simulink model "Lab_6_Hydraulic_Assist_ibrahim"  (R2018b)
settings: Solver=VariableStepAuto  StartTime=0.0  StopTime=5  MaxStep=0.0001  RelTol=1e-3
undefined symbols (not defined in the file): a_neg, A_neg, A_pos, a_pos, ar_neg, Ar_neg, Ar_pos, ar_pos, F_human_max, F_rated_wheel, k, k_dec, kr, kr_dec, Lever_ratio, P_servo_max, R_master, R_servo, R_wheel, s_rated_wheel, V_initial
libraries: nesl_utility x16, sdl_lib x9, fl_lib x8, eeGeneralControl x1, SignalEditorBlockLib x1
settings Model: Creator=AHMED MOHSEN  LastModifiedBy=AHMED MOHSEN
settings DataIOCC: ReturnWorkspaceOutputs=on
settings DebuggingCC: UnconnectedInputMsg=none  UnconnectedOutputMsg=none  UnconnectedLineMsg=none
settings ModelReferenceCC: EnableRefExpFcnMdlSchedulingChecks=off
settings RTWCC: Description=Generic Real-Time Target

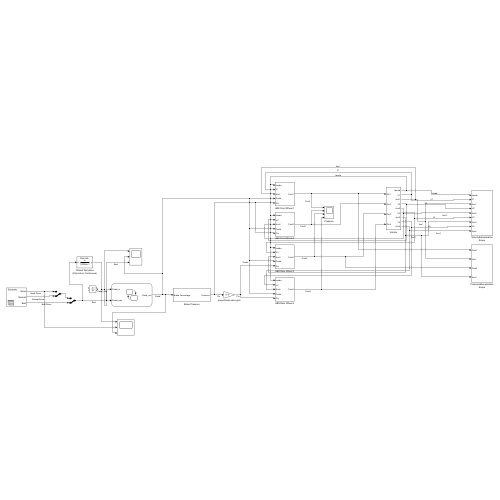
[thumbnail: Simulink's stored preview of the top-level diagram]
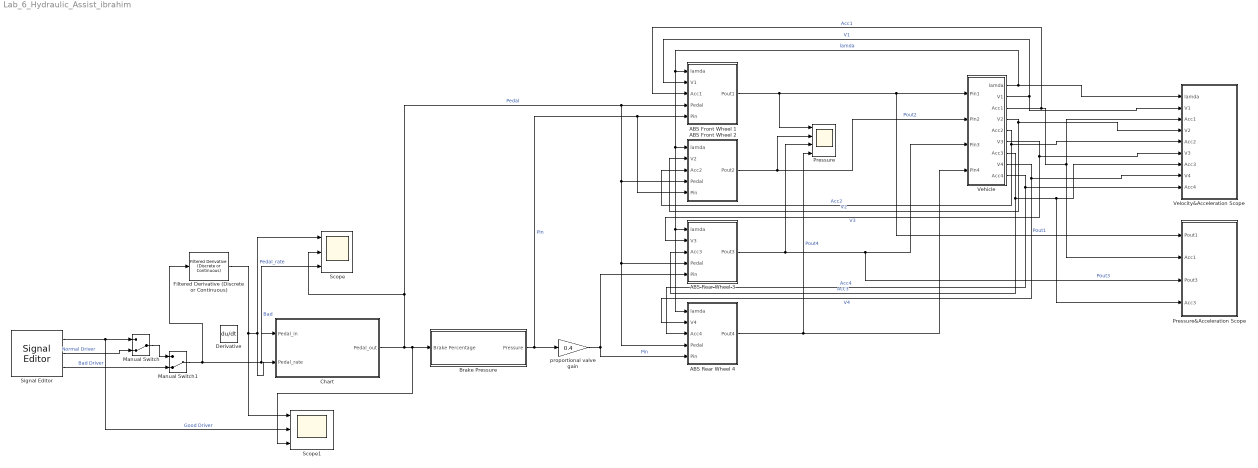
== system Lab_6_Hydraulic_Assist_ibrahim ==
  ABS Front Wheel 1 : Subsystem
  ABS Front Wheel 2 : Subsystem
  ABS Rear Wheel 3 : Subsystem
  ABS Rear Wheel 4 : Subsystem
  Brake Pressure : Subsystem
  Chart : Stateflow chart  TreatAsAtomicUnit=on
  Derivative : Derivative
  Filtered Derivative (Discrete or Continuous) : eeGeneralControl/Filtered Derivative (Discrete or Continuous)  K=1  T=0.002  B=inf  A=-inf  minRatio=10  init_option=Inherited from block input  x0=0  Ts=-1
  Manual Switch : ManualSwitch  CurrentSetting=0
  Manual Switch1 : ManualSwitch  CurrentSetting=0
  Pressure : Scope  NumInputPorts=4
  Pressure&Acceleration Scope : Subsystem
  Scope : Scope  NumInputPorts=3
  Scope1 : Scope  NumInputPorts=3
  Signal Editor : SignalEditorBlockLib/Signal Editor  FileName=D:\College\Senior 2 Mechatronics\Second Term\Introduction to Automotive\Report 6 lab\scenario2.mat  ActiveScenario=Scenario  ActiveSignal=Good  IsBus=off  OutputBusObjectStr=Bus: BusObject  SampleTime=0  Interpolate=off  ZeroCross=off  OutputAfterFinalValue=Setting to zero  Unit=inherit
  Vehicle : Subsystem
  Velocity&Acceleration Scope : Subsystem
  proportional valve gain : Gain  Gain=0.4
  wires:
  Signal Editor/1 -> Scope1/2, Manual Switch/1  "Good Driver"
  Signal Editor/2 -> Manual Switch/2  "Normal Driver"
  Signal Editor/3 -> Manual Switch1/2  "Bad Driver"
  Manual Switch/1 -> Manual Switch1/1
  Manual Switch1/1 -> Filtered Derivative (Discrete or Continuous)/1, Scope/3, Chart/1(Pedal_in)  "Bad"
  Vehicle/5(Acc2) -> Velocity&Acceleration Scope/5(Acc2), ABS Front Wheel 2/3(Acc2)  "Acc2"
  Vehicle/8(V4) -> Velocity&Acceleration Scope/8(V4), ABS Rear Wheel 4/2(V4)  "V4"
  Vehicle/6(V3) -> ABS Rear Wheel 3/2(V3), Velocity&Acceleration Scope/6(V3)  "V3"
  Vehicle/4(V2) -> ABS Front Wheel 2/2(V2), Velocity&Acceleration Scope/4(V2)  "V2"
  Vehicle/7(Acc3) -> Velocity&Acceleration Scope/7(Acc3), Pressure&Acceleration Scope/4(Acc3), ABS Rear Wheel 3/3(Acc3)  "Acc3"
  Vehicle/9(Acc4) -> Velocity&Acceleration Scope/9(Acc4), ABS Rear Wheel 4/3(Acc4)  "Acc4"
  ABS Rear Wheel 3/1(Pout3) -> Pressure/3, Pressure&Acceleration Scope/3(Pout3), Vehicle/3(Pin3)  "Pout3"
  ABS Rear Wheel 4/1(Pout4) -> Pressure/4, Vehicle/4(Pin4)  "Pout4"
  Chart/1(Pedal_out) -> Scope1/3, Brake Pressure/1(Brake Percentage), Scope/2, ABS Rear Wheel 4/4(Pedal), ABS Rear Wheel 3/4(Pedal), ABS Front Wheel 2/4(Pedal), ABS Front Wheel 1/4(Pedal)  "Pedal"
  Vehicle/1(lamda) -> Velocity&Acceleration Scope/1(lamda), ABS Rear Wheel 4/1(lamda), ABS Rear Wheel 3/1(lamda), ABS Front Wheel 2/1(lamda), ABS Front Wheel 1/1(lamda)  "lamda"
  ABS Front Wheel 1/1(Pout1) -> Pressure/1, Pressure&Acceleration Scope/1(Pout1), Vehicle/1(Pin1)  "Pout1"
  ABS Front Wheel 2/1(Pout2) -> Pressure/2, Vehicle/2(Pin2)  "Pout2"
  Brake Pressure/1(Pressure) -> proportional valve gain/1, ABS Front Wheel 2/5(Pin), ABS Front Wheel 1/5(Pin)  "Pin"
  Vehicle/3(Acc1) -> Pressure&Acceleration Scope/2(Acc1), Velocity&Acceleration Scope/3(Acc1), ABS Front Wheel 1/3(Acc1)  "Acc1"
  proportional valve gain/1 -> ABS Rear Wheel 4/5(Pin), ABS Rear Wheel 3/5(Pin)  "Pin"
  Vehicle/2(V1) -> ABS Front Wheel 1/2(V1), Velocity&Acceleration Scope/2(V1)  "V1"
  Filtered Derivative (Discrete or Continuous)/1 -> Scope1/1, Scope/1, Chart/2(Pedal_rate)  "Pedal_rate"

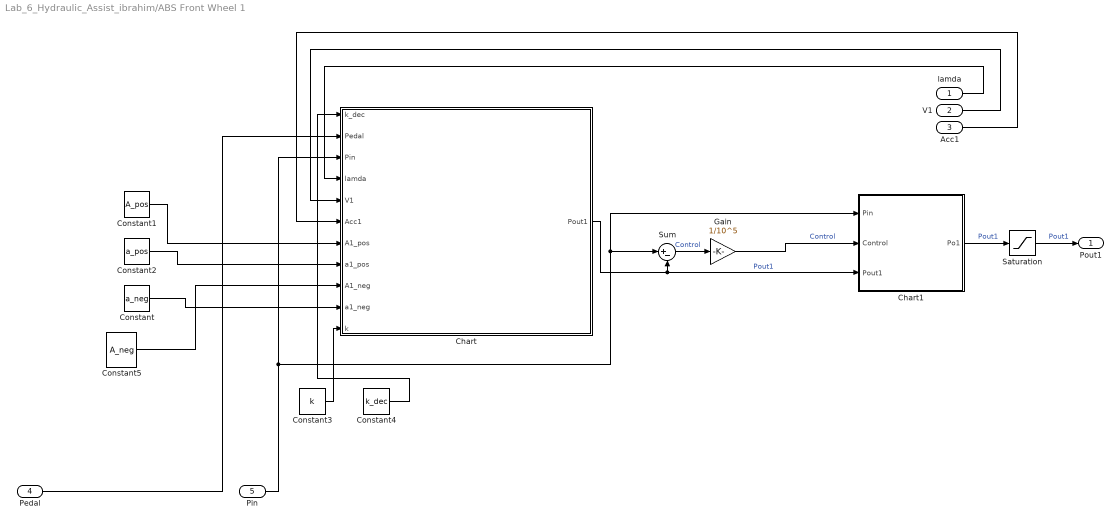
== system Lab_6_Hydraulic_Assist_ibrahim/ABS Front Wheel 1 ==
  lamda : Inport
  V1 : Inport  Port=2
  Acc1 : Inport  Port=3
  Pedal : Inport  Port=4
  Pin : Inport  Port=5
  Chart : Stateflow chart  TreatAsAtomicUnit=on
  Chart1 : Stateflow chart  TreatAsAtomicUnit=on
  Constant : Constant  Value=a_neg
  Constant1 : Constant  Value=A_pos
  Constant2 : Constant  Value=a_pos
  Constant3 : Constant  Value=k
  Constant4 : Constant  Value=k_dec
  Constant5 : Constant  Value=A_neg
  Gain : Gain  Gain=1/10^5
  Saturation : Saturate  UpperLimit=inf  LowerLimit=0
  Sum : Sum  Inputs=|+-
  Pout1 : Outport
  wires:
  Pin/1 -> Chart1/1(Pin), Sum/1, Chart/3(Pin)
  Acc1/1 -> Chart/6(Acc1)
  Pedal/1 -> Chart/2(Pedal)
  Constant2/1 -> Chart/8(a1_pos)
  Sum/1 -> Gain/1  "Control"
  lamda/1 -> Chart/4(lamda)
  Constant/1 -> Chart/10(a1_neg)
  Chart/1(Pout1) -> Chart1/3(Pout1), Sum/2  "Pout1"
  Constant1/1 -> Chart/7(A1_pos)
  Chart1/1(Po1) -> Saturation/1  "Pout1"
  V1/1 -> Chart/5(V1)
  Constant3/1 -> Chart/11(k)
  Gain/1 -> Chart1/2(Control)  "Control"
  Constant4/1 -> Chart/1(k_dec)
  Constant5/1 -> Chart/9(A1_neg)
  Saturation/1 -> Pout1/1  "Pout1"

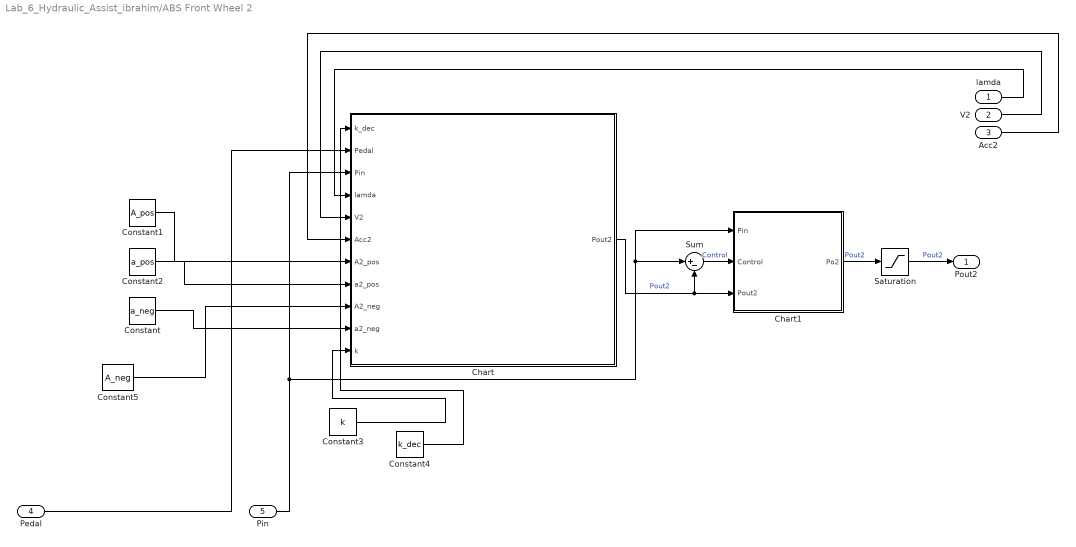
== system Lab_6_Hydraulic_Assist_ibrahim/ABS Front Wheel 2 ==
  lamda : Inport
  V2 : Inport  Port=2
  Acc2 : Inport  Port=3
  Pedal : Inport  Port=4
  Pin : Inport  Port=5
  Chart : Stateflow chart  TreatAsAtomicUnit=on
  Chart1 : Stateflow chart  TreatAsAtomicUnit=on
  Constant : Constant  Value=a_neg
  Constant1 : Constant  Value=A_pos
  Constant2 : Constant  Value=a_pos
  Constant3 : Constant  Value=k
  Constant4 : Constant  Value=k_dec
  Constant5 : Constant  Value=A_neg
  Saturation : Saturate  UpperLimit=inf  LowerLimit=0
  Sum : Sum  Inputs=|+-
  Pout2 : Outport
  wires:
  Pin/1 -> Chart1/1(Pin), Sum/1, Chart/3(Pin)
  Acc2/1 -> Chart/6(Acc2)
  Pedal/1 -> Chart/2(Pedal)
  Constant2/1 -> Chart/8(a2_pos)
  Sum/1 -> Chart1/2(Control)  "Control"
  lamda/1 -> Chart/4(lamda)
  Constant/1 -> Chart/10(a2_neg)
  Chart/1(Pout2) -> Chart1/3(Pout2), Sum/2  "Pout2"
  Constant1/1 -> Chart/7(A2_pos)
  Chart1/1(Po2) -> Saturation/1  "Pout2"
  V2/1 -> Chart/5(V2)
  Constant3/1 -> Chart/11(k)
  Constant4/1 -> Chart/1(k_dec)
  Constant5/1 -> Chart/9(A2_neg)
  Saturation/1 -> Pout2/1  "Pout2"

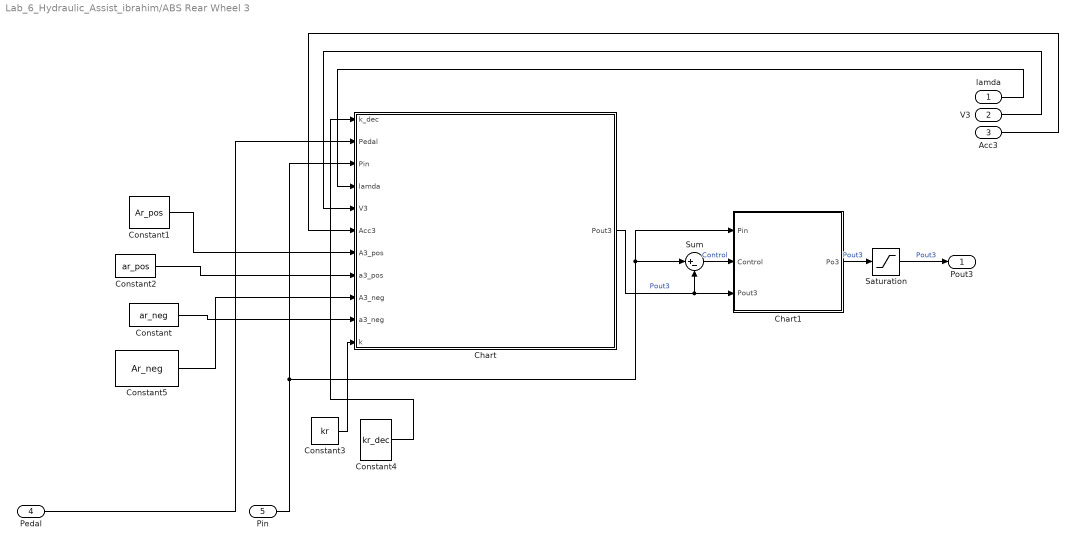
== system Lab_6_Hydraulic_Assist_ibrahim/ABS Rear Wheel 3 ==
  lamda : Inport
  V3 : Inport  Port=2
  Acc3 : Inport  Port=3
  Pedal : Inport  Port=4
  Pin : Inport  Port=5
  Chart : Stateflow chart  TreatAsAtomicUnit=on
  Chart1 : Stateflow chart  TreatAsAtomicUnit=on
  Constant : Constant  Value=ar_neg
  Constant1 : Constant  Value=Ar_pos
  Constant2 : Constant  Value=ar_pos
  Constant3 : Constant  Value=kr
  Constant4 : Constant  Value=kr_dec
  Constant5 : Constant  Value=Ar_neg
  Saturation : Saturate  UpperLimit=inf  LowerLimit=0
  Sum : Sum  Inputs=|+-
  Pout3 : Outport
  wires:
  Pin/1 -> Chart1/1(Pin), Sum/1, Chart/3(Pin)
  Acc3/1 -> Chart/6(Acc3)
  Pedal/1 -> Chart/2(Pedal)
  Constant2/1 -> Chart/8(a3_pos)
  Sum/1 -> Chart1/2(Control)  "Control"
  lamda/1 -> Chart/4(lamda)
  Constant/1 -> Chart/10(a3_neg)
  Chart/1(Pout3) -> Chart1/3(Pout3), Sum/2  "Pout3"
  Constant1/1 -> Chart/7(A3_pos)
  Chart1/1(Po3) -> Saturation/1  "Pout3"
  V3/1 -> Chart/5(V3)
  Constant3/1 -> Chart/11(k)
  Constant4/1 -> Chart/1(k_dec)
  Constant5/1 -> Chart/9(A3_neg)
  Saturation/1 -> Pout3/1  "Pout3"

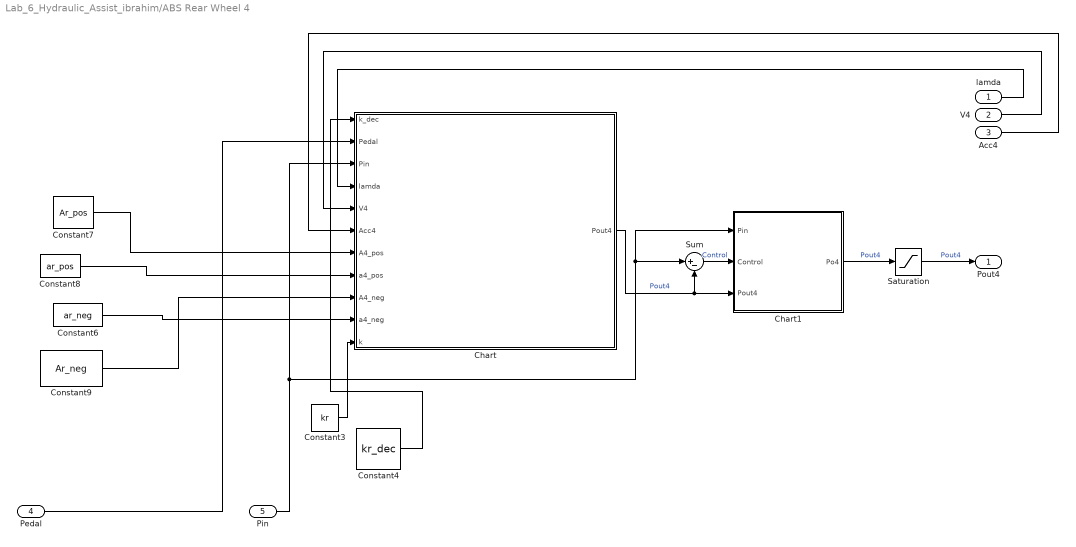
== system Lab_6_Hydraulic_Assist_ibrahim/ABS Rear Wheel 4 ==
  lamda : Inport
  V4 : Inport  Port=2
  Acc4 : Inport  Port=3
  Pedal : Inport  Port=4
  Pin : Inport  Port=5
  Chart : Stateflow chart  TreatAsAtomicUnit=on
  Chart1 : Stateflow chart  TreatAsAtomicUnit=on
  Constant3 : Constant  Value=kr
  Constant4 : Constant  Value=kr_dec
  Constant6 : Constant  Value=ar_neg
  Constant7 : Constant  Value=Ar_pos
  Constant8 : Constant  Value=ar_pos
  Constant9 : Constant  Value=Ar_neg
  Saturation : Saturate  UpperLimit=inf  LowerLimit=0
  Sum : Sum  Inputs=|+-
  Pout4 : Outport
  wires:
  Pin/1 -> Chart1/1(Pin), Sum/1, Chart/3(Pin)
  Acc4/1 -> Chart/6(Acc4)
  Pedal/1 -> Chart/2(Pedal)
  Constant8/1 -> Chart/8(a4_pos)
  Sum/1 -> Chart1/2(Control)  "Control"
  lamda/1 -> Chart/4(lamda)
  Constant6/1 -> Chart/10(a4_neg)
  Chart/1(Pout4) -> Chart1/3(Pout4), Sum/2  "Pout4"
  Constant7/1 -> Chart/7(A4_pos)
  Chart1/1(Po4) -> Saturation/1  "Pout4"
  V4/1 -> Chart/5(V4)
  Constant3/1 -> Chart/11(k)
  Constant4/1 -> Chart/1(k_dec)
  Constant9/1 -> Chart/9(A4_neg)
  Saturation/1 -> Pout4/1  "Pout4"

== system Lab_6_Hydraulic_Assist_ibrahim/Brake Pressure ==
  Brake Percentage : Inport
  Add : Sum
  booster (pressure*area) : Gain  Gain=P_servo_max*pi*(R_servo)^2
  human force : Gain  Gain=F_human_max
  master /area of master : Gain  Gain=1/(pi*(R_master)^2)
  mechanical adv lever (pedal) : Gain  Gain=Lever_ratio
  Pressure : Outport
  wires:
  human force/1 -> mechanical adv lever (pedal)/1
  Brake Percentage/1 -> human force/1, booster (pressure*area)/1
  mechanical adv lever (pedal)/1 -> Add/1
  Add/1 -> master /area of master/1
  master /area of master/1 -> Pressure/1  "pressure"
  booster (pressure*area)/1 -> Add/2

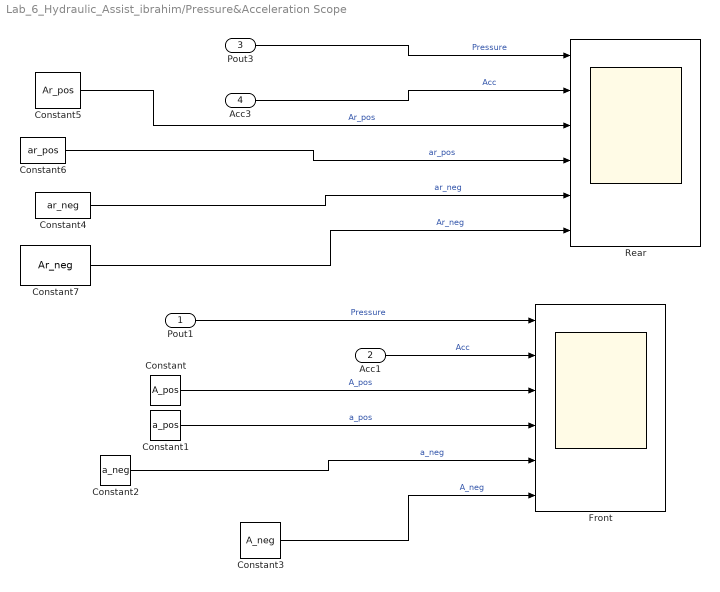
== system Lab_6_Hydraulic_Assist_ibrahim/Pressure&Acceleration Scope ==
  Pout1 : Inport
  Acc1 : Inport  Port=2
  Pout3 : Inport  Port=3
  Acc3 : Inport  Port=4
  Constant : Constant  Value=A_pos
  Constant1 : Constant  Value=a_pos
  Constant2 : Constant  Value=a_neg
  Constant3 : Constant  Value=A_neg
  Constant4 : Constant  Value=ar_neg
  Constant5 : Constant  Value=Ar_pos
  Constant6 : Constant  Value=ar_pos
  Constant7 : Constant  Value=Ar_neg
  Front : Scope  NumInputPorts=6
  Rear : Scope  NumInputPorts=6
  wires:
  Constant1/1 -> Front/4  "a_pos"
  Pout3/1 -> Rear/1  "Pressure"
  Constant/1 -> Front/3  "A_pos"
  Constant3/1 -> Front/6  "A_neg"
  Acc3/1 -> Rear/2  "Acc"
  Constant2/1 -> Front/5  "a_neg"
  Pout1/1 -> Front/1  "Pressure"
  Acc1/1 -> Front/2  "Acc"
  Constant7/1 -> Rear/6  "Ar_neg"
  Constant4/1 -> Rear/5  "ar_neg"
  Constant6/1 -> Rear/4  "ar_pos"
  Constant5/1 -> Rear/3  "Ar_pos"

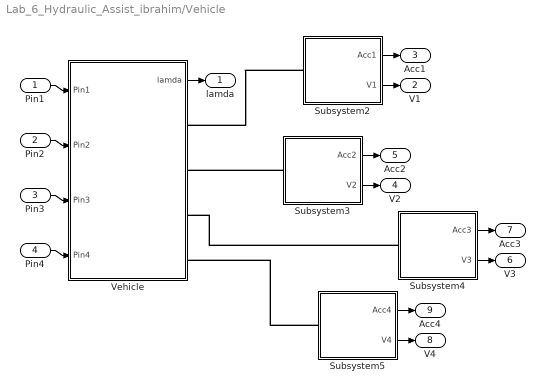
== system Lab_6_Hydraulic_Assist_ibrahim/Vehicle ==
  Pin1 : Inport
  Pin2 : Inport  Port=2
  Pin3 : Inport  Port=3
  Pin4 : Inport  Port=4
  Subsystem2 : Subsystem
  Subsystem3 : Subsystem
  Subsystem4 : Subsystem
  Subsystem5 : Subsystem
  Vehicle : Subsystem
  lamda : Outport
  V1 : Outport  Port=2
  Acc1 : Outport  Port=3
  V2 : Outport  Port=4
  Acc2 : Outport  Port=5
  V3 : Outport  Port=6
  Acc3 : Outport  Port=7
  V4 : Outport  Port=8
  Acc4 : Outport  Port=9
  wires:
  Subsystem2/1(Acc1) -> Acc1/1
  Pin4/1 -> Vehicle/4(Pin4)
  Pin2/1 -> Vehicle/2(Pin2)
  Pin1/1 -> Vehicle/1(Pin1)
  Pin3/1 -> Vehicle/3(Pin3)
  Subsystem2/2(V1) -> V1/1
  Subsystem5/1(Acc4) -> Acc4/1
  Subsystem3/1(Acc2) -> Acc2/1
  Subsystem3/2(V2) -> V2/1
  Vehicle/1(lamda) -> lamda/1
  Subsystem5/2(V4) -> V4/1
  Subsystem4/1(Acc3) -> Acc3/1
  Subsystem4/2(V3) -> V3/1
  connections:
  Subsystem5/LConn1 -- Vehicle/RConn4
  Subsystem4/LConn1 -- Vehicle/RConn3
  Subsystem2/LConn1 -- Vehicle/RConn1
  Subsystem3/LConn1 -- Vehicle/RConn2

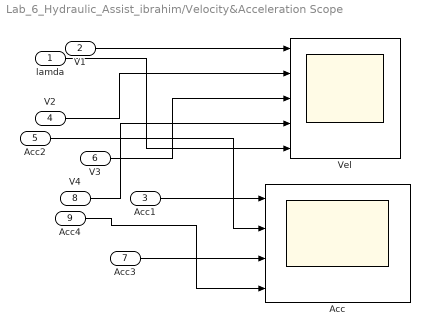
== system Lab_6_Hydraulic_Assist_ibrahim/Velocity&Acceleration Scope ==
  lamda : Inport
  V1 : Inport  Port=2
  Acc1 : Inport  Port=3
  V2 : Inport  Port=4
  Acc2 : Inport  Port=5
  V3 : Inport  Port=6
  Acc3 : Inport  Port=7
  V4 : Inport  Port=8
  Acc4 : Inport  Port=9
  Acc : Scope  NumInputPorts=4
  Vel : Scope  NumInputPorts=5
  wires:
  Acc3/1 -> Acc/3
  lamda/1 -> Vel/5
  V3/1 -> Vel/3
  Acc1/1 -> Acc/1
  Acc4/1 -> Acc/4
  Acc2/1 -> Acc/2
  V1/1 -> Vel/1
  V4/1 -> Vel/4
  V2/1 -> Vel/2

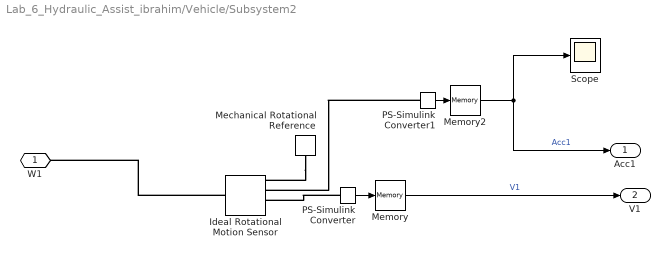
== system Lab_6_Hydraulic_Assist_ibrahim/Vehicle/Subsystem2 ==
  Ideal Rotational Motion Sensor : fl_lib/Mechanical/Mechanical Sensors/Ideal Rotational Motion Sensor  reference=foundation.enum.MeasurementReference.difference  acceleration_port=true  velocity_port=true  position_port=true  wrap_angle=false  offset=0 rad
      settings: InternalSimscapePortConfiguration="{\"Bottom\":[],\"Left\":[{\"id\":\"R\",\"label\":\"R\",\"type\":\"foundation.mechanical.rotational.rotational\"}],\"Right\":[{\"id\":\"C\",\"label\":\"C\",\"type\":\"foundation.mechanical.rotational.rotational\"},{\"id\":\"alpha\",\"label\":\"α\",\"type\":\"output\"},{\"id\":\"W\",\"label\":\"W\",\"type\":\"output\"},{\"id\":\"A\",\"label\":\"A\",\"type\":\"output\"}],\"Top\":[]}"
  Mechanical Rotational Reference : fl_lib/Mechanical/Rotational Elements/Mechanical Rotational Reference
  Memory : Memory  InitialCondition=V_initial/3.6/R_wheel  InheritSampleTime=on
  Memory2 : Memory  InheritSampleTime=on
  PS-Simulink Converter : nesl_utility/PS-Simulink Converter  PhysicalDomain=network_engine_domain  SubClassName=ps_output  LeftPortType=input  RightPortType=output  PseudoPeriodic=off  Frequencies=[]  VectorFormat=inherit  Unit=rad/s  AffineConversion=off
  PS-Simulink Converter1 : nesl_utility/PS-Simulink Converter  PhysicalDomain=network_engine_domain  SubClassName=ps_output  LeftPortType=input  RightPortType=output  PseudoPeriodic=off  Frequencies=[]  VectorFormat=inherit  Unit=rad/s^2  AffineConversion=off
  Scope : Scope
  W1 : PMIOPort  Side=Left
  Acc1 : Outport
  V1 : Outport  Port=2
  wires:
  Memory/1 -> V1/1  "V1"
  PS-Simulink Converter/1 -> Memory/1
  PS-Simulink Converter1/1 -> Memory2/1
  Memory2/1 -> Acc1/1, Scope/1  "Acc1"
  connections:
  Ideal Rotational Motion Sensor/LConn1 -- W1/RConn1
  PS-Simulink Converter/LConn1 -- Ideal Rotational Motion Sensor/RConn3
  Mechanical Rotational Reference/LConn1 -- Ideal Rotational Motion Sensor/RConn1
  PS-Simulink Converter1/LConn1 -- Ideal Rotational Motion Sensor/RConn2

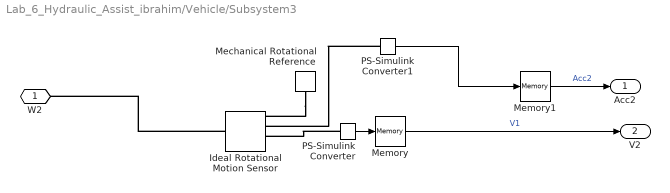
== system Lab_6_Hydraulic_Assist_ibrahim/Vehicle/Subsystem3 ==
  Ideal Rotational Motion Sensor : fl_lib/Mechanical/Mechanical Sensors/Ideal Rotational Motion Sensor  reference=foundation.enum.MeasurementReference.difference  acceleration_port=true  velocity_port=true  position_port=true  wrap_angle=false  offset=0 rad
      settings: InternalSimscapePortConfiguration="{\"Bottom\":[],\"Left\":[{\"id\":\"R\",\"label\":\"R\",\"type\":\"foundation.mechanical.rotational.rotational\"}],\"Right\":[{\"id\":\"C\",\"label\":\"C\",\"type\":\"foundation.mechanical.rotational.rotational\"},{\"id\":\"alpha\",\"label\":\"α\",\"type\":\"output\"},{\"id\":\"W\",\"label\":\"W\",\"type\":\"output\"},{\"id\":\"A\",\"label\":\"A\",\"type\":\"output\"}],\"Top\":[]}"
  Mechanical Rotational Reference : fl_lib/Mechanical/Rotational Elements/Mechanical Rotational Reference
  Memory : Memory  InitialCondition=V_initial/3.6/R_wheel  InheritSampleTime=on
  Memory1 : Memory  InheritSampleTime=on
  PS-Simulink Converter : nesl_utility/PS-Simulink Converter  PhysicalDomain=network_engine_domain  SubClassName=ps_output  LeftPortType=input  RightPortType=output  PseudoPeriodic=off  Frequencies=[]  VectorFormat=inherit  Unit=rad/s  AffineConversion=off
  PS-Simulink Converter1 : nesl_utility/PS-Simulink Converter  PhysicalDomain=network_engine_domain  SubClassName=ps_output  LeftPortType=input  RightPortType=output  PseudoPeriodic=off  Frequencies=[]  VectorFormat=inherit  Unit=rad/s^2  AffineConversion=off
  W2 : PMIOPort  Side=Left
  Acc2 : Outport
  V2 : Outport  Port=2
  wires:
  Memory/1 -> V2/1  "V1"
  PS-Simulink Converter/1 -> Memory/1
  PS-Simulink Converter1/1 -> Memory1/1
  Memory1/1 -> Acc2/1  "Acc2"
  connections:
  Ideal Rotational Motion Sensor/LConn1 -- W2/RConn1
  PS-Simulink Converter/LConn1 -- Ideal Rotational Motion Sensor/RConn3
  Mechanical Rotational Reference/LConn1 -- Ideal Rotational Motion Sensor/RConn1
  PS-Simulink Converter1/LConn1 -- Ideal Rotational Motion Sensor/RConn2

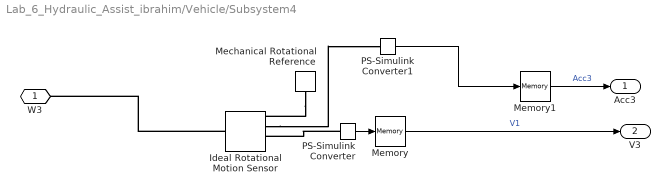
== system Lab_6_Hydraulic_Assist_ibrahim/Vehicle/Subsystem4 ==
  Ideal Rotational Motion Sensor : fl_lib/Mechanical/Mechanical Sensors/Ideal Rotational Motion Sensor  reference=foundation.enum.MeasurementReference.difference  acceleration_port=true  velocity_port=true  position_port=true  wrap_angle=false  offset=0 rad
      settings: InternalSimscapePortConfiguration="{\"Bottom\":[],\"Left\":[{\"id\":\"R\",\"label\":\"R\",\"type\":\"foundation.mechanical.rotational.rotational\"}],\"Right\":[{\"id\":\"C\",\"label\":\"C\",\"type\":\"foundation.mechanical.rotational.rotational\"},{\"id\":\"alpha\",\"label\":\"α\",\"type\":\"output\"},{\"id\":\"W\",\"label\":\"W\",\"type\":\"output\"},{\"id\":\"A\",\"label\":\"A\",\"type\":\"output\"}],\"Top\":[]}"
  Mechanical Rotational Reference : fl_lib/Mechanical/Rotational Elements/Mechanical Rotational Reference
  Memory : Memory  InitialCondition=V_initial/3.6/R_wheel  InheritSampleTime=on
  Memory1 : Memory  InheritSampleTime=on
  PS-Simulink Converter : nesl_utility/PS-Simulink Converter  PhysicalDomain=network_engine_domain  SubClassName=ps_output  LeftPortType=input  RightPortType=output  PseudoPeriodic=off  Frequencies=[]  VectorFormat=inherit  Unit=rad/s  AffineConversion=off
  PS-Simulink Converter1 : nesl_utility/PS-Simulink Converter  PhysicalDomain=network_engine_domain  SubClassName=ps_output  LeftPortType=input  RightPortType=output  PseudoPeriodic=off  Frequencies=[]  VectorFormat=inherit  Unit=rad/s^2  AffineConversion=off
  W3 : PMIOPort  Side=Left
  Acc3 : Outport
  V3 : Outport  Port=2
  wires:
  Memory/1 -> V3/1  "V1"
  PS-Simulink Converter/1 -> Memory/1
  PS-Simulink Converter1/1 -> Memory1/1
  Memory1/1 -> Acc3/1  "Acc3"
  connections:
  Ideal Rotational Motion Sensor/LConn1 -- W3/RConn1
  PS-Simulink Converter/LConn1 -- Ideal Rotational Motion Sensor/RConn3
  Mechanical Rotational Reference/LConn1 -- Ideal Rotational Motion Sensor/RConn1
  Ideal Rotational Motion Sensor/RConn2 -- PS-Simulink Converter1/LConn1

== system Lab_6_Hydraulic_Assist_ibrahim/Vehicle/Subsystem5 ==
  Ideal Rotational Motion Sensor : fl_lib/Mechanical/Mechanical Sensors/Ideal Rotational Motion Sensor  reference=foundation.enum.MeasurementReference.difference  acceleration_port=true  velocity_port=true  position_port=true  wrap_angle=false  offset=0 rad
      settings: InternalSimscapePortConfiguration="{\"Bottom\":[],\"Left\":[{\"id\":\"R\",\"label\":\"R\",\"type\":\"foundation.mechanical.rotational.rotational\"}],\"Right\":[{\"id\":\"C\",\"label\":\"C\",\"type\":\"foundation.mechanical.rotational.rotational\"},{\"id\":\"alpha\",\"label\":\"α\",\"type\":\"output\"},{\"id\":\"W\",\"label\":\"W\",\"type\":\"output\"},{\"id\":\"A\",\"label\":\"A\",\"type\":\"output\"}],\"Top\":[]}"
  Mechanical Rotational Reference : fl_lib/Mechanical/Rotational Elements/Mechanical Rotational Reference
  Memory : Memory  InitialCondition=V_initial/3.6/R_wheel  InheritSampleTime=on
  Memory1 : Memory  InheritSampleTime=on
  PS-Simulink Converter : nesl_utility/PS-Simulink Converter  PhysicalDomain=network_engine_domain  SubClassName=ps_output  LeftPortType=input  RightPortType=output  PseudoPeriodic=off  Frequencies=[]  VectorFormat=inherit  Unit=rad/s  AffineConversion=off
  PS-Simulink Converter1 : nesl_utility/PS-Simulink Converter  PhysicalDomain=network_engine_domain  SubClassName=ps_output  LeftPortType=input  RightPortType=output  PseudoPeriodic=off  Frequencies=[]  VectorFormat=inherit  Unit=rad/s^2  AffineConversion=off
  W4 : PMIOPort  Side=Left
  Acc4 : Outport
  V4 : Outport  Port=2
  wires:
  Memory/1 -> V4/1  "V1"
  PS-Simulink Converter/1 -> Memory/1
  PS-Simulink Converter1/1 -> Memory1/1
  Memory1/1 -> Acc4/1  "Acc1"
  connections:
  Ideal Rotational Motion Sensor/LConn1 -- W4/RConn1
  PS-Simulink Converter/LConn1 -- Ideal Rotational Motion Sensor/RConn3
  Mechanical Rotational Reference/LConn1 -- Ideal Rotational Motion Sensor/RConn1
  PS-Simulink Converter1/LConn1 -- Ideal Rotational Motion Sensor/RConn2

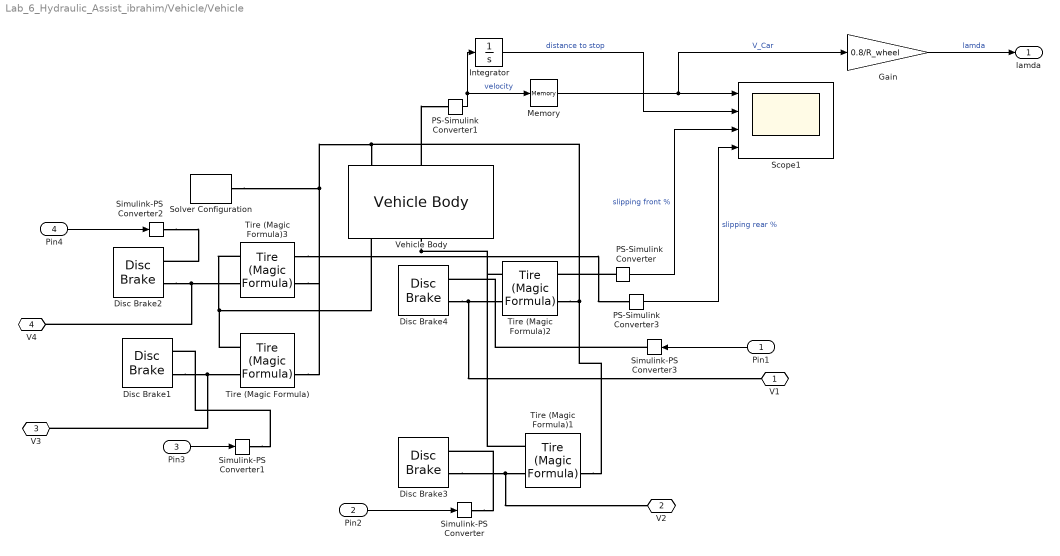
== system Lab_6_Hydraulic_Assist_ibrahim/Vehicle/Vehicle ==
  Pin1 : Inport
  Pin2 : Inport  Port=2
  Pin3 : Inport  Port=3
  Pin4 : Inport  Port=4
  Disc Brake1 : sdl_lib/Brakes & Detents/Rotational/Disc Brake  r_mean=R_disk mm  bore=D_cylinder mm  n_pads=2  thermal_port=simscape.enum.thermaleffects.omit  mu_static=0.9  mu_coulomb=0.7  temperature_TLU=[280, 300, 320] K  mu_static_TLU=[.9, .8, .7]  mu_coulomb_TLU=[.8, .7, .6]  brkwy_vel=0.1 rad/s  visc_coef=Visc_coeff N*m*s/rad  enable_faults=simscape.enum.onoff.off  faulted_pressure=0 bar  external_fault=simscape.enum.onoff.off  temporal_fault=simscape.enum.onoff.off  fault_time=5 s  report_fault=simscape.enum.assert.action.none  thermal_mass=50 kJ/K  temperature_specify=off  temperature_priority=High  temperature=300 K  temperature_nominal_specify=off  temperature_nominal_unit=K  temperature_nominal_value=1
  Disc Brake2 : sdl_lib/Brakes & Detents/Rotational/Disc Brake  r_mean=R_disk mm  bore=D_cylinder mm  n_pads=2  thermal_port=simscape.enum.thermaleffects.omit  mu_static=0.9  mu_coulomb=0.7  temperature_TLU=[280, 300, 320] K  mu_static_TLU=[.9, .8, .7]  mu_coulomb_TLU=[.8, .7, .6]  brkwy_vel=0.1 rad/s  visc_coef=Visc_coeff N*m*s/rad  enable_faults=simscape.enum.onoff.off  faulted_pressure=0 bar  external_fault=simscape.enum.onoff.off  temporal_fault=simscape.enum.onoff.off  fault_time=5 s  report_fault=simscape.enum.assert.action.none  thermal_mass=50 kJ/K  temperature_specify=off  temperature_priority=High  temperature=300 K  temperature_nominal_specify=off  temperature_nominal_unit=K  temperature_nominal_value=1
  Disc Brake3 : sdl_lib/Brakes & Detents/Rotational/Disc Brake  r_mean=R_disk mm  bore=D_cylinder mm  n_pads=2  thermal_port=simscape.enum.thermaleffects.omit  mu_static=0.9  mu_coulomb=0.7  temperature_TLU=[280, 300, 320] K  mu_static_TLU=[.9, .8, .7]  mu_coulomb_TLU=[.8, .7, .6]  brkwy_vel=0.1 rad/s  visc_coef=Visc_coeff N*m*s/rad  enable_faults=simscape.enum.onoff.off  faulted_pressure=0 bar  external_fault=simscape.enum.onoff.off  temporal_fault=simscape.enum.onoff.off  fault_time=5 s  report_fault=simscape.enum.assert.action.none  thermal_mass=50 kJ/K  temperature_specify=off  temperature_priority=High  temperature=300 K  temperature_nominal_specify=off  temperature_nominal_unit=K  temperature_nominal_value=1
  Disc Brake4 : sdl_lib/Brakes & Detents/Rotational/Disc Brake  r_mean=R_disk mm  bore=D_cylinder mm  n_pads=NO_brake_pads  thermal_port=simscape.enum.thermaleffects.omit  mu_static=0.9  mu_coulomb=0.7  temperature_TLU=[280, 300, 320] K  mu_static_TLU=[.9, .8, .7]  mu_coulomb_TLU=[.8, .7, .6]  brkwy_vel=0.1 rad/s  visc_coef=Visc_coeff N*m*s/rad  enable_faults=simscape.enum.onoff.off  faulted_pressure=0 bar  external_fault=simscape.enum.onoff.off  temporal_fault=simscape.enum.onoff.off  fault_time=5 s  report_fault=simscape.enum.assert.action.none  thermal_mass=50 kJ/K  temperature_specify=off  temperature_priority=High  temperature=300 K  temperature_nominal_specify=off  temperature_nominal_unit=K  temperature_nominal_value=1
  Gain : Gain  Gain=0.8/R_wheel
  Integrator : Integrator
  Memory : Memory  InitialCondition=V_initial/3.6
  PS-Simulink Converter : nesl_utility/PS-Simulink Converter  PhysicalDomain=network_engine_domain  SubClassName=ps_output  LeftPortType=input  RightPortType=output  PseudoPeriodic=off  Frequencies=[]  VectorFormat=1-D array  Unit=inherit  AffineConversion=off
  PS-Simulink Converter1 : nesl_utility/PS-Simulink Converter  PhysicalDomain=network_engine_domain  SubClassName=ps_output  LeftPortType=input  RightPortType=output  PseudoPeriodic=off  Frequencies=[]  VectorFormat=inherit  Unit=m/s  AffineConversion=off
  PS-Simulink Converter3 : nesl_utility/PS-Simulink Converter  PhysicalDomain=network_engine_domain  SubClassName=ps_output  LeftPortType=input  RightPortType=output  PseudoPeriodic=off  Frequencies=[]  VectorFormat=1-D array  Unit=inherit  AffineConversion=off
  Scope1 : Scope  NumInputPorts=4
  Simulink-PS Converter{,1..3} (4 alike) : nesl_utility/Simulink-PS Converter  PhysicalDomain=network_engine_domain  SubClassName=ps_input  LeftPortType=input  RightPortType=output  PseudoPeriodic=off  Frequencies=[]  NoiseDistribution=none  NoiseParameters=[]  Unit=Pa  AffineConversion=off  FilteringAndDerivatives=provide  SimscapeFilterOrder=1  InputFilterTimeConstant=0.001  UdotUserProvided=0
  Solver Configuration : nesl_utility/Solver Configuration  PhysicalDomain=network_engine_domain  SubClassName=solver  LeftPortType=input  RightPortType=generic  Tones=[]  Harmonics=[]  SimulateNoise=off  Profile=off  UseLocalSampling=off  EnableSwitchedLinearOptims=on  FrequencyDomain=off  UseCCode=off  RelTol=0.001  AbsTol=0.001  MinStep=1e-09  ToWorkspace=off  RevertToSquareIcSolve=off  NumHomotopyIterations=100  PhasorMode=off  PhasorModeNumHarmonics=1  ConsistencySolver=NEWTON_XTOL_AFTER_FTOL  IndexReductionMethod=DerivativeReplacement  DoDC=off  ResidualTolerance=1e-09  ConsistencyTolSource=GLOBAL  ConsistencyAbsTol=0.001  ConsistencyRelTol=0.001  ConsistencyTolFactor=0.001  UseLocalSolver=off  LocalSolverChoice=NE_BACKWARD_EULER_ADVANCER  ResolveIndetEquations=on  FunctionEvalNumThread=1  LocalSolverSampleTime=0.001  DoFixedCost=off  MaxNonlinIter=3  MaxModeIter=2  ComputeImpulses=off  ImpulseIterations=2  LinearAlgebra=auto  LinearAlgebraNumThread=0  EquationFormulation=NE_TIME_EF  DelaysMemoryBudget=1024  AutomaticFiltering=on  FilteringTimeConstant=0.001  PartitionStorageMethod=AS_NEEDED  PartitionMemoryBudget=1024  PartitionMethod=ROBUST  MultibodyUseLocalSolver=off  MultibodyLocalSolverChoice=ODE1  MultibodyLocalSolverSampleTime=0.001
  Tire (Magic Formula){,1..3} (4 alike) : sdl_lib/Tires & Vehicles/Tire (Magic Formula)  parameterization=sdl.enum.magic_tire_model.peak  F_z1=F_rated_wheel N  F_x1=F_rated_wheel*s_rated_wheel N  kappa1=10  B_m=10  C_m=1.9  D_m=1  E_m=0.97  fz0=4000 N  p_Cx=1.685  p_Dx=[1.21, -.037]  p_Ex=[.344, .095, -.02, 0]  p_Kx=[21.51, -.163, .245]  p_Hx=[-.002, .002]  p_Vx=[0, 0]  rolling_radius_model=sdl.enum.RollingRadiusParameterization.Constant  r_e=R_wheel m  r_0=0.3 m  breff=8.39  dreff=0.26  freff=0.074  q_re0=0.99  q_v1=0.008  longvl=17 m/s  cz=5e5 N/m  model_resistance=false  resistance_model=sdl.enum.rollingResistanceParameterization.constant  coeff=0.015  p_tire=250e3 Pa  alpha=-0.003  beta=0.97  coeff_a=84e-4  coeff_b=6.2e-4 s/m  coeff_c=1.6e-4 s^2/m^2  p_tire0=240e3 Pa  fz0_resistance=4000 N  vH0=16 m/s  q_Sy=[.0082, 0, .0014, .001, 0, 0, 1.08, -.5]  v_thr=0.001 m/s  enable_scaling_coefficients=false  lfzO=1  lcx=1  lmux=1  lex=1  lkx=1  lhx=1  lvx=1  lmy=1  model_compliance=sdl.enum.compliance.off  stiffness=1e6 N/m  damping=1000 N*s/m  model_inertia=sdl.enum.model_inertia.on  inertia=1 kg*m^2  initial_velocity=V_initial/3.6/R_wheel rad/s  vxlow=1 m/s  v_tr_thr=0.1 m/s  kpumin=-1.5  kpumax=1.5
  Vehicle Body : sdl_lib/Tires & Vehicles/Vehicle Body  mass=m_vehicle kg  n_w=2  x_f=f_CG m  x_r=r_CG m  y_c=h_CG m  mass_var=simscape.enum.onoff.off  g=9.81 m/s^2  liftoff_warning=simscape.enum.onoff.off  area=3 m^2  Cd=Drag_coeff  rho=1.18 kg/m^3  model_pitch=simscape.enum.onoff.off  inertia=4000 kg*m^2  suspension_model=sdl.enum.linearTLU.linear  k_f=1e4 N/m  b_f=1e4 N*s/m  k_r=1e4 N/m  b_r=1e4 N*s/m  k_f_TLU=[-2000, -1000, 0, 1000, 2000] N  x_f_TLU=[-.4, -.2, 0, .2, .4] m  b_f_TLU=[-200, -100, 0, 100, 200] N  v_f_TLU=[-4, -2, 0, 2, 4] m/s  k_r_TLU=[-2000, -1000, 0, 1000, 2000] N  x_r_TLU=[-.4, -.2, 0, .2, .4] m  b_r_TLU=[-200, -100, 0, 100, 200] N  v_r_TLU=[-4, -2, 0, 2, 4] m/s  interp_method=simscape.enum.interpolation.linear  extrap_method=simscape.enum.extrapolation.linear  model_hardstop=simscape.enum.onoff.off  upper_bound_f=.25 m  lower_bound_f=-.25 m  stop_k_f=1e6 N/m  stop_b_f=150 N*s/m  upper_bound_r=.25 m  lower_bound_r=-.25 m  stop_k_r=1e6 N/m  stop_b_r=150 N*s/m  initial_pitch=0 rad  initial_pitch_rate=0 rad/s  v_specify=on  v_priority=High  v=V_initial kph  v_nominal_specify=off  v_nominal_unit=m/s  v_nominal_value=1
  V1 : PMIOPort  Side=Right
  V2 : PMIOPort  Port=2  Side=Right
  V3 : PMIOPort  Port=3  Side=Right
  V4 : PMIOPort  Port=4  Side=Right
  lamda : Outport
  wires:
  Memory/1 -> Gain/1, Scope1/1  "V_Car"
  PS-Simulink Converter1/1 -> Integrator/1, Memory/1  "velocity"
  Pin2/1 -> Simulink-PS Converter/1
  Pin3/1 -> Simulink-PS Converter1/1
  Integrator/1 -> Scope1/2  "distance to stop"
  PS-Simulink Converter/1 -> Scope1/3  "slipping front %"
  PS-Simulink Converter3/1 -> Scope1/4  "slipping rear %"
  Pin4/1 -> Simulink-PS Converter2/1
  Gain/1 -> lamda/1  "lamda"
  Pin1/1 -> Simulink-PS Converter3/1
  connections:
  Tire (Magic Formula)2/RConn2 -- Tire (Magic Formula)1/RConn2 -- Tire (Magic Formula)/RConn2 -- Tire (Magic Formula)3/RConn2 -- Solver Configuration/RConn1 -- Vehicle Body/LConn1
  Disc Brake1/LConn2 -- V3/RConn1 -- Tire (Magic Formula)/LConn2
  Vehicle Body/LConn2 -- PS-Simulink Converter1/LConn1
  Tire (Magic Formula)/LConn1 -- Tire (Magic Formula)3/LConn1 -- Vehicle Body/RConn1
  PS-Simulink Converter/LConn1 -- Tire (Magic Formula)2/RConn1
  Disc Brake4/LConn2 -- V1/RConn1 -- Tire (Magic Formula)2/LConn2
  Disc Brake3/LConn2 -- V2/RConn1 -- Tire (Magic Formula)1/LConn2
  Simulink-PS Converter2/RConn1 -- Disc Brake2/LConn1
  Disc Brake2/LConn2 -- V4/RConn1 -- Tire (Magic Formula)3/LConn2
  Vehicle Body/RConn2 -- Tire (Magic Formula)1/LConn1 -- Tire (Magic Formula)2/LConn1
  Simulink-PS Converter1/RConn1 -- Disc Brake1/LConn1
  Tire (Magic Formula)3/RConn1 -- PS-Simulink Converter3/LConn1
  Simulink-PS Converter/RConn1 -- Disc Brake3/LConn1
  Simulink-PS Converter3/RConn1 -- Disc Brake4/LConn1

== stateflow chart Lab_6_Hydraulic_Assist_ibrahim/ABS Front Wheel 1/Chart1 ==
  state start
    during:
    Po1=Pout1
  state limit
    during:
    Po1=Pin
  (default) -> start
  start -> limit : [Control<0]
  limit -> start : [Control>0 | Control==0]
  data: Pin input; Control input; Pout1 input; Po1 output

== stateflow chart Lab_6_Hydraulic_Assist_ibrahim/ABS Front Wheel 2/Chart ==
  state hold
    during:
    Pout2=Pout2
  state start
    Pout2=Pin
  state inc
    during:
    Pout2=Pout2+k
  state dec
    during:
    Pout2=Pout2-k_dec
  hold -> start [order 1] : [Pedal<0.02]
  start -> hold : [Pedal>0.55]
  hold -> inc [order 3] : [Acc2<a2_pos && Acc2>a2_neg]
  (default) -> start
  inc -> hold [order 2] : [Acc2<a2_neg && Acc2>A2_neg]
  inc -> start [order 1] : [Pedal<0.02]
  dec -> start [order 1] : [Pedal<0.02]
  hold -> inc [order 2] : [Acc2>A2_pos]
  inc -> hold [order 3] : [Acc2<A2_pos && Acc2>a2_pos]
  hold -> dec [order 4] : [Acc2<A2_neg]
  dec -> hold [order 2] : [Acc2>a2_neg && Acc2<A2_pos]
  data: k_dec input; Pedal input; Pin input; lamda input; V2 input; Acc2 input; Pout2 output; A2_pos input; a2_pos input; A2_neg input; a2_neg input; k input; data local

== stateflow chart Lab_6_Hydraulic_Assist_ibrahim/ABS Front Wheel 1/Chart ==
  state hold
    during:
    Pout1=Pout1
  state start
    Pout1=Pin
  state inc
    during:
    Pout1=Pout1+k
  state dec
    during:
    Pout1=Pout1-k_dec
  hold -> start [order 1] : [Pedal<0.02]
  start -> hold : [Pedal>0.55]
  hold -> inc [order 4] : [Acc1<a1_pos && Acc1>a1_neg]
  (default) -> start
  inc -> hold [order 2] : [Acc1<a1_neg && Acc1>A1_neg]
  inc -> start [order 1] : [Pedal<0.02]
  dec -> start [order 1] : [Pedal<0.02]
  hold -> inc [order 3] : [Acc1>A1_pos]
  inc -> hold [order 3] : [Acc1<A1_pos && Acc1>a1_pos]
  dec -> hold [order 2] : [Acc1>a1_neg && Acc1<A1_pos]
  hold -> dec [order 2] : [Acc1<A1_neg]
  data: k_dec input; Pedal input; Pin input; lamda input; V1 input; Acc1 input; Pout1 output; A1_pos input; a1_pos input; A1_neg input; a1_neg input; k input; r local =10^4

== stateflow chart Lab_6_Hydraulic_Assist_ibrahim/ABS Front Wheel 2/Chart1 ==
  state start
    during:
    Po2=Pout2
  state limit
    during:
    Po2=Pin
  (default) -> start
  start -> limit : [Control<0]
  limit -> start : [Control>0 | Control==0]
  data: Pin input; Control input; Pout2 input; Po2 output

== stateflow chart Lab_6_Hydraulic_Assist_ibrahim/ABS Rear Wheel 3/Chart ==
  state hold
    during:
    Pout3=Pout3
  state start
    Pout3=Pin
  state inc
    during:
    Pout3=Pout3+k
  state dec
    during:
    Pout3=Pout3-k_dec
  hold -> start [order 1] : [Pedal<0.02]
  start -> hold : [Pedal>0.55]
  hold -> inc [order 4] : [Acc3<a3_pos && Acc3>a3_neg]
  (default) -> start
  inc -> hold [order 2] : [Acc3<a3_neg && Acc3>A3_neg]
  inc -> start [order 1] : [Pedal<0.02]
  dec -> start [order 1] : [Pedal<0.02]
  hold -> inc [order 3] : [Acc3>A3_pos]
  inc -> hold [order 3] : [Acc3<A3_pos && Acc3>a3_pos]
  hold -> dec [order 2] : [Acc3<A3_neg]
  dec -> hold [order 2] : [Acc3>a3_neg && Acc3<A3_pos]
  data: k_dec input; Pedal input; Pin input; lamda input; V3 input; Acc3 input; Pout3 output; A3_pos input; a3_pos input; A3_neg input; a3_neg input; k input; r local =10^4

== stateflow chart Lab_6_Hydraulic_Assist_ibrahim/ABS Rear Wheel 3/Chart1 ==
  state start
    during:
    Po3=Pout3
  state limit
    during:
    Po3=Pin
  (default) -> start
  start -> limit : [Control<0]
  limit -> start : [Control>0 | Control==0]
  data: Pin input; Control input; Pout3 input; Po3 output

== stateflow chart Lab_6_Hydraulic_Assist_ibrahim/ABS Rear Wheel 4/Chart ==
  state hold
    during:
    Pout4=Pout4
  state start
    Pout4=Pin
  state inc
    during:
    Pout4=Pout4+k
  state dec
    during:
    Pout4=Pout4-k_dec
  hold -> start [order 1] : [Pedal<0.02]
  start -> hold : [Pedal>0.55]
  hold -> inc [order 3] : [Acc4<a4_pos && Acc4>a4_neg]
  (default) -> start
  inc -> hold [order 2] : [Acc4<a4_neg && Acc4>A4_neg]
  inc -> start [order 1] : [Pedal<0.02]
  hold -> inc [order 2] : [Acc4>A4_pos]
  dec -> start [order 1] : [Pedal<0.02]
  inc -> hold [order 3] : [Acc4<A4_pos && Acc4>a4_pos]
  hold -> dec [order 4] : [Acc4<A4_neg]
  dec -> hold [order 2] : [Acc4>a4_neg && Acc4<A4_pos]
  data: k_dec input; Pedal input; Pin input; lamda input; V4 input; Acc4 input; Pout4 output; A4_pos input; a4_pos input; A4_neg input; a4_neg input; k input; r local =10^4

== stateflow chart Lab_6_Hydraulic_Assist_ibrahim/ABS Rear Wheel 4/Chart1 ==
  state start
    during:
    Po4=Pout4
  state limit
    during:
    Po4=Pin
  (default) -> start
  start -> limit : [Control<0]
  limit -> start : [Control>0 | Control==0]
  data: Pin input; Control input; Pout4 input; Po4 output

== stateflow chart Lab_6_Hydraulic_Assist_ibrahim/Chart ==
  state Passive
    during:
    Pedal_out=Pedal_in;
  state Active
    during:
    Pedal_out=1;
  (default) -> Passive
  Passive -> Active : [Pedal_rate>0.99]
  Active -> Passive : [Pedal_rate<0.01]
  data: Pedal_in input; Pedal_rate input; Pedal_out output
